simulink model "Buck_closedloop"  (R2022a)
settings: Solver=ode45  StartTime=0.0  StopTime=0.01  RelTol=1e-3  EnableMultiTasking=on
settings Model: Creator=Landon  LastModifiedBy=mluser
settings SolverCC: AlgebraicLoopSolver=TrustRegion
settings DataIOCC: LimitDataPoints=on  SaveFormat=Array  ReturnWorkspaceOutputs=off
settings OptimizationCC: LifeSpan=inf
settings DebuggingCC: UnconnectedInputMsg=warning  UnconnectedOutputMsg=warning  UnconnectedLineMsg=warning  SFUnexpectedBacktrackingDiag=warning  SFNoUnconditionalDefaultTransitionDiag=warning  SFExecutionAtInitializationDiag=none  SFMachineParentedDataDiag=warning  ArithmeticOperatorsInVariantConditions=warning
settings HardwareCC: ProdBitPerPointer=32  ProdBitPerSizeT=32  ProdBitPerPtrDiffT=32  ProdLargestAtomicFloat=None  ProdIntDivRoundTo=Undefined  ProdEndianess=Unspecified  ProdWordSize=32  ProdHWDeviceType=32-bit Generic
settings ModelReferenceCC: PropagateSignalLabelsOutOfModel=off
settings SFSimCC: SimUseLocalCustomCode=off  CustomCodeUndefinedFunction=UseInterfaceOnly
settings RTWCC: RTWUseLocalCustomCode=off
settings CodeAppCC: StateflowObjectComments=on
settings GRTTargetCC: TargetLangStandard=C89/C90 (ANSI)
settings ConfigComp: CovMetricSettings=dw  CovSaveCumulativeToWorkspaceVar=on  CovSaveSingleToWorkspaceVar=on  CovExternalEMLEnable=off

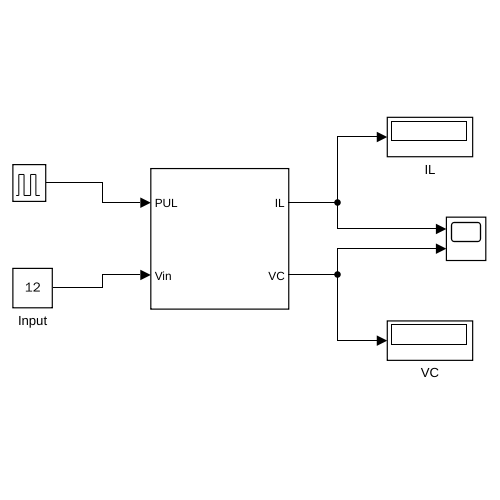
[thumbnail: Simulink's stored preview of the top-level diagram]
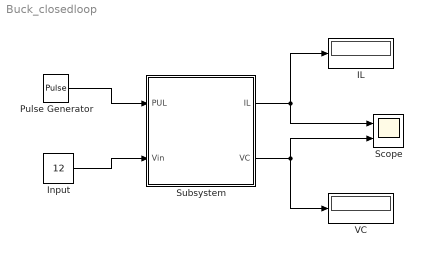
== system Buck_closedloop ==
  IL : Display
  Input : Constant  Value=12
  Pulse Generator : DiscretePulseGenerator  PulseType=Time based  Period=1/5000  PulseWidth=.25*100
  Scope : Scope  NumInputPorts=2
  Subsystem : Subsystem
  VC : Display
  wires:
  Subsystem/2(VC) -> Scope/2, VC/1
  Subsystem/1(IL) -> Scope/1, IL/1
  Pulse Generator/1 -> Subsystem/1(PUL)
  Input/1 -> Subsystem/2(Vin)

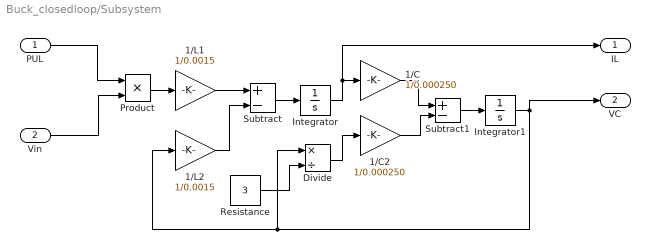
== system Buck_closedloop/Subsystem ==
  PUL : Inport
  Vin : Inport  Port=2
  1/C : Gain  Gain=1/0.000250
  1/C2 : Gain  Gain=1/0.000250
  1/L1 : Gain  Gain=1/0.0015
  1/L2 : Gain  Gain=1/0.0015
  Divide : Product  Inputs=*/
  Integrator : Integrator
  Integrator1 : Integrator
  Product : Product
  Resistance : Constant  Value=3
  Subtract : Sum  Inputs=+-
  Subtract1 : Sum  Inputs=+-
  IL : Outport
  VC : Outport  Port=2
  wires:
  PUL/1 -> Product/1
  Subtract1/1 -> Integrator1/1
  Integrator1/1 -> VC/1, 1/L2/1, Divide/1
  Resistance/1 -> Divide/2
  Vin/1 -> Product/2
  Product/1 -> 1/L1/1
  Subtract/1 -> Integrator/1
  1/C/1 -> Subtract1/1
  1/L1/1 -> Subtract/1
  1/L2/1 -> Subtract/2
  1/C2/1 -> Subtract1/2
  Divide/1 -> 1/C2/1
  Integrator/1 -> IL/1, 1/C/1
